simulink model "gm_uz_pmsm_model_6ph_dqxy"  (R2024b)
settings: Solver=FixedStepAuto  StartTime=0.0  StopTime=0.5  RelTol=1e-3
PreLoadFcn:
  | uz_pmsm_model_6ph_dqxy_init_parameter
undefined symbols (not defined in the file or in its folder): friction_coefficient, inertia, k_i_d, k_i_x, k_i_y, k_p_d, k_p_q, k_p_x, k_p_y, L_d, L_q, L_x, L_y, polepair, psi_pm, R_1, setpoint_step, simulate_mechanical, simulate_open_loop, static_friction_torque
libraries: hdlmdlgenlib x5, slpidlib x4
(part 2 of 2)

== system gm_uz_pmsm_model_6ph_dqxy/uz_pmsm_model/Data Type Conversion18 ==
  In1 : Inport
  Data Type Conversion18 : DataTypeConversion  OutDataTypeStr=double  RndMeth=Nearest  SampleTime=1e-08  SaturateOnIntegerOverflow=off
  Data Type Conversion18_pd1 : Delay  DelayLength=3
  Out1 : Outport
  wires:
  In1/1 -> Data Type Conversion18/1
  Data Type Conversion18/1 -> Data Type Conversion18_pd1/1
  Data Type Conversion18_pd1/1 -> Out1/1

== system gm_uz_pmsm_model_6ph_dqxy/uz_pmsm_model/Data Type Conversion19 ==
  In1 : Inport
  Data Type Conversion19 : DataTypeConversion  OutDataTypeStr=double  RndMeth=Nearest  SampleTime=1e-08  SaturateOnIntegerOverflow=off
  Data Type Conversion19_pd1 : Delay  DelayLength=3
  Out1 : Outport
  wires:
  In1/1 -> Data Type Conversion19/1
  Data Type Conversion19/1 -> Data Type Conversion19_pd1/1
  Data Type Conversion19_pd1/1 -> Out1/1

== system gm_uz_pmsm_model_6ph_dqxy/uz_pmsm_model/Data Type Conversion2 ==
  In1 : Inport
  Data Type Conversion2 : DataTypeConversion  OutDataTypeStr=double  RndMeth=Nearest  SampleTime=1e-08  SaturateOnIntegerOverflow=off
  Data Type Conversion2_pd1 : Delay  DelayLength=3
  Out1 : Outport
  wires:
  In1/1 -> Data Type Conversion2/1
  Data Type Conversion2/1 -> Data Type Conversion2_pd1/1
  Data Type Conversion2_pd1/1 -> Out1/1

== system gm_uz_pmsm_model_6ph_dqxy/uz_pmsm_model/Data Type Conversion20 ==
  In1 : Inport
  Data Type Conversion20 : DataTypeConversion  OutDataTypeStr=double  RndMeth=Nearest  SampleTime=1e-08  SaturateOnIntegerOverflow=off
  Data Type Conversion20_pd1 : Delay  DelayLength=3
  Out1 : Outport
  wires:
  In1/1 -> Data Type Conversion20/1
  Data Type Conversion20/1 -> Data Type Conversion20_pd1/1
  Data Type Conversion20_pd1/1 -> Out1/1

== system gm_uz_pmsm_model_6ph_dqxy/uz_pmsm_model/Data Type Conversion21 ==
  In1 : Inport
  Data Type Conversion21 : DataTypeConversion  OutDataTypeStr=single  RndMeth=Nearest  SampleTime=1e-08  SaturateOnIntegerOverflow=off
  Data Type Conversion21_pd1 : Delay  DelayLength=3
  Out1 : Outport
  wires:
  In1/1 -> Data Type Conversion21/1
  Data Type Conversion21/1 -> Data Type Conversion21_pd1/1
  Data Type Conversion21_pd1/1 -> Out1/1

== system gm_uz_pmsm_model_6ph_dqxy/uz_pmsm_model/Data Type Conversion22 ==
  In1 : Inport
  Data Type Conversion22 : DataTypeConversion  OutDataTypeStr=single  RndMeth=Nearest  SampleTime=1e-08  SaturateOnIntegerOverflow=off
  Data Type Conversion22_pd1 : Delay  DelayLength=3
  Out1 : Outport
  wires:
  In1/1 -> Data Type Conversion22/1
  Data Type Conversion22/1 -> Data Type Conversion22_pd1/1
  Data Type Conversion22_pd1/1 -> Out1/1

== system gm_uz_pmsm_model_6ph_dqxy/uz_pmsm_model/Data Type Conversion3 ==
  In1 : Inport
  Data Type Conversion3 : DataTypeConversion  OutDataTypeStr=double  RndMeth=Nearest  SampleTime=1e-08  SaturateOnIntegerOverflow=off
  Data Type Conversion3_pd1 : Delay  DelayLength=3
  Out1 : Outport
  wires:
  In1/1 -> Data Type Conversion3/1
  Data Type Conversion3/1 -> Data Type Conversion3_pd1/1
  Data Type Conversion3_pd1/1 -> Out1/1

== system gm_uz_pmsm_model_6ph_dqxy/uz_pmsm_model/Data Type Conversion4 ==
  In1 : Inport
  Data Type Conversion4 : DataTypeConversion  OutDataTypeStr=double  RndMeth=Nearest  SampleTime=1e-08  SaturateOnIntegerOverflow=off
  Data Type Conversion4_pd1 : Delay  DelayLength=3
  Out1 : Outport
  wires:
  In1/1 -> Data Type Conversion4/1
  Data Type Conversion4/1 -> Data Type Conversion4_pd1/1
  Data Type Conversion4_pd1/1 -> Out1/1

== system gm_uz_pmsm_model_6ph_dqxy/uz_pmsm_model/Data Type Conversion5 ==
  In1 : Inport
  Data Type Conversion5 : DataTypeConversion  OutDataTypeStr=double  RndMeth=Nearest  SampleTime=1e-08  SaturateOnIntegerOverflow=off
  Data Type Conversion5_pd1 : Delay  DelayLength=3
  Out1 : Outport
  wires:
  In1/1 -> Data Type Conversion5/1
  Data Type Conversion5/1 -> Data Type Conversion5_pd1/1
  Data Type Conversion5_pd1/1 -> Out1/1

== system gm_uz_pmsm_model_6ph_dqxy/uz_pmsm_model/Data Type Conversion6 ==
  In1 : Inport
  Data Type Conversion6 : DataTypeConversion  OutDataTypeStr=double  RndMeth=Nearest  SampleTime=1e-08  SaturateOnIntegerOverflow=off
  Data Type Conversion6_pd1 : Delay  DelayLength=3
  Out1 : Outport
  wires:
  In1/1 -> Data Type Conversion6/1
  Data Type Conversion6/1 -> Data Type Conversion6_pd1/1
  Data Type Conversion6_pd1/1 -> Out1/1

== system gm_uz_pmsm_model_6ph_dqxy/uz_pmsm_model/Data Type Conversion7 ==
  In1 : Inport
  Data Type Conversion7 : DataTypeConversion  OutDataTypeStr=double  RndMeth=Nearest  SampleTime=1e-08  SaturateOnIntegerOverflow=off
  Data Type Conversion7_pd1 : Delay  DelayLength=3
  Out1 : Outport
  wires:
  In1/1 -> Data Type Conversion7/1
  Data Type Conversion7/1 -> Data Type Conversion7_pd1/1
  Data Type Conversion7_pd1/1 -> Out1/1

== system gm_uz_pmsm_model_6ph_dqxy/uz_pmsm_model/Data Type Conversion8 ==
  In1 : Inport
  Data Type Conversion8 : DataTypeConversion  OutDataTypeStr=double  RndMeth=Nearest  SampleTime=1e-08  SaturateOnIntegerOverflow=off
  Data Type Conversion8_pd1 : Delay  DelayLength=3
  Out1 : Outport
  wires:
  In1/1 -> Data Type Conversion8/1
  Data Type Conversion8/1 -> Data Type Conversion8_pd1/1
  Data Type Conversion8_pd1/1 -> Out1/1

== system gm_uz_pmsm_model_6ph_dqxy/uz_pmsm_model/Data Type Conversion9 ==
  In1 : Inport
  Data Type Conversion9 : DataTypeConversion  OutDataTypeStr=double  RndMeth=Nearest  SampleTime=1e-08  SaturateOnIntegerOverflow=off
  Data Type Conversion9_pd1 : Delay  DelayLength=3
  Out1 : Outport
  wires:
  In1/1 -> Data Type Conversion9/1
  Data Type Conversion9/1 -> Data Type Conversion9_pd1/1
  Data Type Conversion9_pd1/1 -> Out1/1

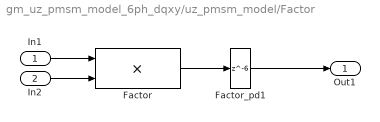
== system gm_uz_pmsm_model_6ph_dqxy/uz_pmsm_model/Factor ==
  In1 : Inport
  In2 : Inport  Port=2
  Factor : Product  Inputs=**  OutDataTypeStr=double  SampleTime=1e-08
  Factor_pd1 : Delay  DelayLength=6
  Out1 : Outport
  wires:
  In1/1 -> Factor/1
  In2/1 -> Factor/2
  Factor/1 -> Factor_pd1/1
  Factor_pd1/1 -> Out1/1

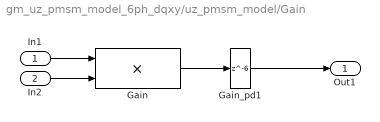
== system gm_uz_pmsm_model_6ph_dqxy/uz_pmsm_model/Gain ==
  In1 : Inport
  In2 : Inport  Port=2
  Gain : Product  Inputs=**  OutDataTypeStr=double  SampleTime=1e-08
  Gain_pd1 : Delay  DelayLength=6
  Out1 : Outport
  wires:
  In1/1 -> Gain/1
  In2/1 -> Gain/2
  Gain/1 -> Gain_pd1/1
  Gain_pd1/1 -> Out1/1

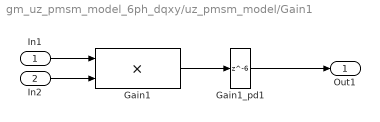
== system gm_uz_pmsm_model_6ph_dqxy/uz_pmsm_model/Gain1 ==
  In1 : Inport
  In2 : Inport  Port=2
  Gain1 : Product  Inputs=**  OutDataTypeStr=double  SampleTime=1e-08
  Gain1_pd1 : Delay  DelayLength=6
  Out1 : Outport
  wires:
  In1/1 -> Gain1/1
  In2/1 -> Gain1/2
  Gain1/1 -> Gain1_pd1/1
  Gain1_pd1/1 -> Out1/1

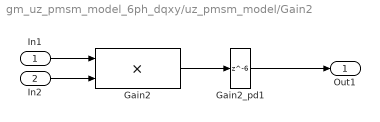
== system gm_uz_pmsm_model_6ph_dqxy/uz_pmsm_model/Gain2 ==
  In1 : Inport
  In2 : Inport  Port=2
  Gain2 : Product  Inputs=**  OutDataTypeStr=double  SampleTime=1e-08
  Gain2_pd1 : Delay  DelayLength=6
  Out1 : Outport
  wires:
  In1/1 -> Gain2/1
  In2/1 -> Gain2/2
  Gain2/1 -> Gain2_pd1/1
  Gain2_pd1/1 -> Out1/1

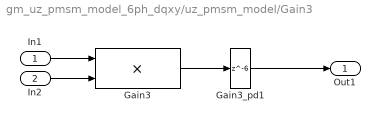
== system gm_uz_pmsm_model_6ph_dqxy/uz_pmsm_model/Gain3 ==
  In1 : Inport
  In2 : Inport  Port=2
  Gain3 : Product  Inputs=**  OutDataTypeStr=double  SampleTime=1e-08
  Gain3_pd1 : Delay  DelayLength=6
  Out1 : Outport
  wires:
  In1/1 -> Gain3/1
  In2/1 -> Gain3/2
  Gain3/1 -> Gain3_pd1/1
  Gain3_pd1/1 -> Out1/1

== system gm_uz_pmsm_model_6ph_dqxy/uz_pmsm_model/Gain4 ==
  In1 : Inport
  In2 : Inport  Port=2
  Gain4 : Product  Inputs=**  OutDataTypeStr=double  SampleTime=1e-08
  Gain4_pd1 : Delay  DelayLength=6
  Out1 : Outport
  wires:
  In1/1 -> Gain4/1
  In2/1 -> Gain4/2
  Gain4/1 -> Gain4_pd1/1
  Gain4_pd1/1 -> Out1/1

== system gm_uz_pmsm_model_6ph_dqxy/uz_pmsm_model/Product ==
  In1 : Inport
  In2 : Inport  Port=2
  Product : Product  Inputs=**  OutDataTypeStr=double  SampleTime=1e-08
  Product_pd1 : Delay  DelayLength=6
  Out1 : Outport
  wires:
  In1/1 -> Product/1
  In2/1 -> Product/2
  Product/1 -> Product_pd1/1
  Product_pd1/1 -> Out1/1

== system gm_uz_pmsm_model_6ph_dqxy/uz_pmsm_model/Product1 ==
  In1 : Inport
  In2 : Inport  Port=2
  Product1 : Product  Inputs=**  OutDataTypeStr=double  SampleTime=1e-08
  Product1_pd1 : Delay  DelayLength=6
  Out1 : Outport
  wires:
  In1/1 -> Product1/1
  In2/1 -> Product1/2
  Product1/1 -> Product1_pd1/1
  Product1_pd1/1 -> Out1/1

== system gm_uz_pmsm_model_6ph_dqxy/uz_pmsm_model/Product10 ==
  In1 : Inport
  In2 : Inport  Port=2
  Product10 : Product  Inputs=**  OutDataTypeStr=double  SampleTime=1e-08
  Product10_pd1 : Delay  DelayLength=6
  Out1 : Outport
  wires:
  In1/1 -> Product10/1
  In2/1 -> Product10/2
  Product10/1 -> Product10_pd1/1
  Product10_pd1/1 -> Out1/1

== system gm_uz_pmsm_model_6ph_dqxy/uz_pmsm_model/Product11 ==
  In1 : Inport
  In2 : Inport  Port=2
  Product11 : Product  Inputs=**  OutDataTypeStr=double  SampleTime=1e-08
  Product11_pd1 : Delay  DelayLength=6
  Out1 : Outport
  wires:
  In1/1 -> Product11/1
  In2/1 -> Product11/2
  Product11/1 -> Product11_pd1/1
  Product11_pd1/1 -> Out1/1

== system gm_uz_pmsm_model_6ph_dqxy/uz_pmsm_model/Product111 ==
  In1 : Inport
  In2 : Inport  Port=2
  Product111 : Product  Inputs=**  OutDataTypeStr=double  SampleTime=1e-08
  Product111_pd1 : Delay  DelayLength=6
  Out1 : Outport
  wires:
  In1/1 -> Product111/1
  In2/1 -> Product111/2
  Product111/1 -> Product111_pd1/1
  Product111_pd1/1 -> Out1/1

== system gm_uz_pmsm_model_6ph_dqxy/uz_pmsm_model/Product12 ==
  In1 : Inport
  In2 : Inport  Port=2
  Product12 : Product  Inputs=**  OutDataTypeStr=double  SampleTime=1e-08
  Product12_pd1 : Delay  DelayLength=6
  Out1 : Outport
  wires:
  In1/1 -> Product12/1
  In2/1 -> Product12/2
  Product12/1 -> Product12_pd1/1
  Product12_pd1/1 -> Out1/1

== system gm_uz_pmsm_model_6ph_dqxy/uz_pmsm_model/Product121 ==
  In1 : Inport
  In2 : Inport  Port=2
  Product121 : Product  Inputs=**  OutDataTypeStr=double  SampleTime=1e-08
  Product121_pd1 : Delay  DelayLength=6
  Out1 : Outport
  wires:
  In1/1 -> Product121/1
  In2/1 -> Product121/2
  Product121/1 -> Product121_pd1/1
  Product121_pd1/1 -> Out1/1

== system gm_uz_pmsm_model_6ph_dqxy/uz_pmsm_model/Product13 ==
  In1 : Inport
  In2 : Inport  Port=2
  Product13 : Product  Inputs=**  OutDataTypeStr=double  SampleTime=1e-08
  Product13_pd1 : Delay  DelayLength=6
  Out1 : Outport
  wires:
  In1/1 -> Product13/1
  In2/1 -> Product13/2
  Product13/1 -> Product13_pd1/1
  Product13_pd1/1 -> Out1/1

== system gm_uz_pmsm_model_6ph_dqxy/uz_pmsm_model/Product2 ==
  In1 : Inport
  In2 : Inport  Port=2
  Product2 : Product  Inputs=**  OutDataTypeStr=double  SampleTime=1e-08
  Product2_pd1 : Delay  DelayLength=6
  Out1 : Outport
  wires:
  In1/1 -> Product2/1
  In2/1 -> Product2/2
  Product2/1 -> Product2_pd1/1
  Product2_pd1/1 -> Out1/1

== system gm_uz_pmsm_model_6ph_dqxy/uz_pmsm_model/Product21 ==
  In1 : Inport
  In2 : Inport  Port=2
  Product21 : Product  Inputs=**  OutDataTypeStr=double  SampleTime=1e-08
  Product21_pd1 : Delay  DelayLength=6
  Out1 : Outport
  wires:
  In1/1 -> Product21/1
  In2/1 -> Product21/2
  Product21/1 -> Product21_pd1/1
  Product21_pd1/1 -> Out1/1

== system gm_uz_pmsm_model_6ph_dqxy/uz_pmsm_model/Product3 ==
  In1 : Inport
  In2 : Inport  Port=2
  Product3 : Product  Inputs=**  OutDataTypeStr=double  SampleTime=1e-08
  Product3_pd1 : Delay  DelayLength=6
  Out1 : Outport
  wires:
  In1/1 -> Product3/1
  In2/1 -> Product3/2
  Product3/1 -> Product3_pd1/1
  Product3_pd1/1 -> Out1/1

== system gm_uz_pmsm_model_6ph_dqxy/uz_pmsm_model/Product31 ==
  In1 : Inport
  In2 : Inport  Port=2
  Product31 : Product  Inputs=**  OutDataTypeStr=double  SampleTime=1e-08
  Product31_pd1 : Delay  DelayLength=6
  Out1 : Outport
  wires:
  In1/1 -> Product31/1
  In2/1 -> Product31/2
  Product31/1 -> Product31_pd1/1
  Product31_pd1/1 -> Out1/1

== system gm_uz_pmsm_model_6ph_dqxy/uz_pmsm_model/Product4 ==
  In1 : Inport
  In2 : Inport  Port=2
  Product4 : Product  Inputs=**  OutDataTypeStr=double  SampleTime=1e-08
  Product4_pd1 : Delay  DelayLength=6
  Out1 : Outport
  wires:
  In1/1 -> Product4/1
  In2/1 -> Product4/2
  Product4/1 -> Product4_pd1/1
  Product4_pd1/1 -> Out1/1

== system gm_uz_pmsm_model_6ph_dqxy/uz_pmsm_model/Product5 ==
  In1 : Inport
  In2 : Inport  Port=2
  Product5 : Product  Inputs=**  OutDataTypeStr=double  SampleTime=1e-08
  Product5_pd1 : Delay  DelayLength=6
  Out1 : Outport
  wires:
  In1/1 -> Product5/1
  In2/1 -> Product5/2
  Product5/1 -> Product5_pd1/1
  Product5_pd1/1 -> Out1/1

== system gm_uz_pmsm_model_6ph_dqxy/uz_pmsm_model/Product6 ==
  In1 : Inport
  In2 : Inport  Port=2
  Product6 : Product  Inputs=**  OutDataTypeStr=double  SampleTime=1e-08
  Product6_pd1 : Delay  DelayLength=6
  Out1 : Outport
  wires:
  In1/1 -> Product6/1
  In2/1 -> Product6/2
  Product6/1 -> Product6_pd1/1
  Product6_pd1/1 -> Out1/1

== system gm_uz_pmsm_model_6ph_dqxy/uz_pmsm_model/Product7 ==
  In1 : Inport
  In2 : Inport  Port=2
  Product7 : Product  Inputs=**  OutDataTypeStr=double  SampleTime=1e-08
  Product7_pd1 : Delay  DelayLength=6
  Out1 : Outport
  wires:
  In1/1 -> Product7/1
  In2/1 -> Product7/2
  Product7/1 -> Product7_pd1/1
  Product7_pd1/1 -> Out1/1

== system gm_uz_pmsm_model_6ph_dqxy/uz_pmsm_model/Product8 ==
  In1 : Inport
  In2 : Inport  Port=2
  Product8 : Product  Inputs=**  OutDataTypeStr=double  SampleTime=1e-08
  Product8_pd1 : Delay  DelayLength=6
  Out1 : Outport
  wires:
  In1/1 -> Product8/1
  In2/1 -> Product8/2
  Product8/1 -> Product8_pd1/1
  Product8_pd1/1 -> Out1/1

== system gm_uz_pmsm_model_6ph_dqxy/uz_pmsm_model/Product9 ==
  In1 : Inport
  In2 : Inport  Port=2
  Product9 : Product  Inputs=**  OutDataTypeStr=double  SampleTime=1e-08
  Product9_pd1 : Delay  DelayLength=6
  Out1 : Outport
  wires:
  In1/1 -> Product9/1
  In2/1 -> Product9/2
  Product9/1 -> Product9_pd1/1
  Product9_pd1/1 -> Out1/1

== system gm_uz_pmsm_model_6ph_dqxy/uz_pmsm_model/Product91 ==
  In1 : Inport
  In2 : Inport  Port=2
  Product91 : Product  Inputs=**  OutDataTypeStr=double  SampleTime=1e-08
  Product91_pd1 : Delay  DelayLength=6
  Out1 : Outport
  wires:
  In1/1 -> Product91/1
  In2/1 -> Product91/2
  Product91/1 -> Product91_pd1/1
  Product91_pd1/1 -> Out1/1

== system gm_uz_pmsm_model_6ph_dqxy/uz_pmsm_model/Sign1 ==
  In1 : Inport
  Sign1 : Signum  SampleTime=1e-08
  Out1 : Outport
  wires:
  In1/1 -> Sign1/1
  Sign1/1 -> Out1/1

== system gm_uz_pmsm_model_6ph_dqxy/uz_pmsm_model/Sum ==
  In1 : Inport
  In2 : Inport  Port=2
  Sum : Sum  Inputs=+-  OutDataTypeStr=double  SampleTime=1e-08
  Sum_pd1 : Delay  DelayLength=6
  Out1 : Outport
  wires:
  In1/1 -> Sum/1
  In2/1 -> Sum/2
  Sum/1 -> Sum_pd1/1
  Sum_pd1/1 -> Out1/1

== system gm_uz_pmsm_model_6ph_dqxy/uz_pmsm_model/Sum1 ==
  In1 : Inport
  In2 : Inport  Port=2
  Sum1 : Sum  Inputs=+-  OutDataTypeStr=double  SampleTime=1e-08
  Sum1_pd1 : Delay  DelayLength=6
  Out1 : Outport
  wires:
  In1/1 -> Sum1/1
  In2/1 -> Sum1/2
  Sum1/1 -> Sum1_pd1/1
  Sum1_pd1/1 -> Out1/1

== system gm_uz_pmsm_model_6ph_dqxy/uz_pmsm_model/Sum1_stage2 ==
  In1 : Inport
  In2 : Inport  Port=2
  Sum1_stage2 : Sum  Inputs=+-  OutDataTypeStr=double  SampleTime=1e-08
  Sum1_stage2_pd1 : Delay  DelayLength=6
  Out1 : Outport
  wires:
  In1/1 -> Sum1_stage2/1
  In2/1 -> Sum1_stage2/2
  Sum1_stage2/1 -> Sum1_stage2_pd1/1
  Sum1_stage2_pd1/1 -> Out1/1

== system gm_uz_pmsm_model_6ph_dqxy/uz_pmsm_model/Sum1_stage3 ==
  In1 : Inport
  In2 : Inport  Port=2
  Sum1_stage3 : Sum  Inputs=+-  OutDataTypeStr=double  SampleTime=1e-08
  Sum1_stage3_pd1 : Delay  DelayLength=6
  Out1 : Outport
  wires:
  In1/1 -> Sum1_stage3/1
  In2/1 -> Sum1_stage3/2
  Sum1_stage3/1 -> Sum1_stage3_pd1/1
  Sum1_stage3_pd1/1 -> Out1/1

== system gm_uz_pmsm_model_6ph_dqxy/uz_pmsm_model/Sum2 ==
  In1 : Inport
  In2 : Inport  Port=2
  Sum2 : Sum  Inputs=+-  OutDataTypeStr=double  SampleTime=1e-08
  Sum2_pd1 : Delay  DelayLength=6
  Out1 : Outport
  wires:
  In1/1 -> Sum2/1
  In2/1 -> Sum2/2
  Sum2/1 -> Sum2_pd1/1
  Sum2_pd1/1 -> Out1/1

== system gm_uz_pmsm_model_6ph_dqxy/uz_pmsm_model/Sum3 ==
  In1 : Inport
  In2 : Inport  Port=2
  Sum3 : Sum  OutDataTypeStr=double  SampleTime=1e-08
  Sum3_pd1 : Delay  DelayLength=6
  Out1 : Outport
  wires:
  In1/1 -> Sum3/1
  In2/1 -> Sum3/2
  Sum3/1 -> Sum3_pd1/1
  Sum3_pd1/1 -> Out1/1

== system gm_uz_pmsm_model_6ph_dqxy/uz_pmsm_model/Sum31 ==
  In1 : Inport
  In2 : Inport  Port=2
  Sum31 : Sum  OutDataTypeStr=double  SampleTime=1e-08
  Sum31_pd1 : Delay  DelayLength=6
  Out1 : Outport
  wires:
  In1/1 -> Sum31/1
  In2/1 -> Sum31/2
  Sum31/1 -> Sum31_pd1/1
  Sum31_pd1/1 -> Out1/1

== system gm_uz_pmsm_model_6ph_dqxy/uz_pmsm_model/Sum32 ==
  In1 : Inport
  In2 : Inport  Port=2
  Sum32 : Sum  OutDataTypeStr=double  SampleTime=1e-08
  Sum32_pd1 : Delay  DelayLength=6
  Out1 : Outport
  wires:
  In1/1 -> Sum32/1
  In2/1 -> Sum32/2
  Sum32/1 -> Sum32_pd1/1
  Sum32_pd1/1 -> Out1/1

== system gm_uz_pmsm_model_6ph_dqxy/uz_pmsm_model/Sum33 ==
  In1 : Inport
  In2 : Inport  Port=2
  Sum33 : Sum  OutDataTypeStr=double  SampleTime=1e-08
  Sum33_pd1 : Delay  DelayLength=6
  Out1 : Outport
  wires:
  In1/1 -> Sum33/1
  In2/1 -> Sum33/2
  Sum33/1 -> Sum33_pd1/1
  Sum33_pd1/1 -> Out1/1

== system gm_uz_pmsm_model_6ph_dqxy/uz_pmsm_model/Sum34 ==
  In1 : Inport
  In2 : Inport  Port=2
  Sum34 : Sum  Inputs=+-  OutDataTypeStr=double  SampleTime=1e-08
  Sum34_pd1 : Delay  DelayLength=6
  Out1 : Outport
  wires:
  In1/1 -> Sum34/1
  In2/1 -> Sum34/2
  Sum34/1 -> Sum34_pd1/1
  Sum34_pd1/1 -> Out1/1

== system gm_uz_pmsm_model_6ph_dqxy/uz_pmsm_model/Sum35 ==
  In1 : Inport
  In2 : Inport  Port=2
  Sum35 : Sum  OutDataTypeStr=double  SampleTime=1e-08
  Sum35_pd1 : Delay  DelayLength=6
  Out1 : Outport
  wires:
  In1/1 -> Sum35/1
  In2/1 -> Sum35/2
  Sum35/1 -> Sum35_pd1/1
  Sum35_pd1/1 -> Out1/1

== system gm_uz_pmsm_model_6ph_dqxy/uz_pmsm_model/Sum3_stage2 ==
  In1 : Inport
  In2 : Inport  Port=2
  Sum3_stage2 : Sum  Inputs=+-  OutDataTypeStr=double  SampleTime=1e-08
  Sum3_stage2_pd1 : Delay  DelayLength=6
  Out1 : Outport
  wires:
  In1/1 -> Sum3_stage2/1
  In2/1 -> Sum3_stage2/2
  Sum3_stage2/1 -> Sum3_stage2_pd1/1
  Sum3_stage2_pd1/1 -> Out1/1

== system gm_uz_pmsm_model_6ph_dqxy/uz_pmsm_model/Sum3_stage3 ==
  In1 : Inport
  In2 : Inport  Port=2
  Sum3_stage3 : Sum  Inputs=+-  OutDataTypeStr=double  SampleTime=1e-08
  Sum3_stage3_pd1 : Delay  DelayLength=6
  Out1 : Outport
  wires:
  In1/1 -> Sum3_stage3/1
  In2/1 -> Sum3_stage3/2
  Sum3_stage3/1 -> Sum3_stage3_pd1/1
  Sum3_stage3_pd1/1 -> Out1/1

== system gm_uz_pmsm_model_6ph_dqxy/uz_pmsm_model/Sum4_stage2 ==
  In1 : Inport
  In2 : Inport  Port=2
  Sum4_stage2 : Sum  OutDataTypeStr=double  SampleTime=1e-08
  Sum4_stage2_pd1 : Delay  DelayLength=6
  Out1 : Outport
  wires:
  In1/1 -> Sum4_stage2/1
  In2/1 -> Sum4_stage2/2
  Sum4_stage2/1 -> Sum4_stage2_pd1/1
  Sum4_stage2_pd1/1 -> Out1/1

== system gm_uz_pmsm_model_6ph_dqxy/uz_pmsm_model/Sum4_stage3 ==
  In1 : Inport
  In2 : Inport  Port=2
  Sum4_stage3 : Sum  Inputs=+-  OutDataTypeStr=double  SampleTime=1e-08
  Sum4_stage3_pd1 : Delay  DelayLength=6
  Out1 : Outport
  wires:
  In1/1 -> Sum4_stage3/1
  In2/1 -> Sum4_stage3/2
  Sum4_stage3/1 -> Sum4_stage3_pd1/1
  Sum4_stage3_pd1/1 -> Out1/1

== system gm_uz_pmsm_model_6ph_dqxy/uz_pmsm_model/Sum5 ==
  In1 : Inport
  In2 : Inport  Port=2
  Sum5 : Sum  OutDataTypeStr=double  SampleTime=1e-08
  Sum5_pd1 : Delay  DelayLength=6
  Out1 : Outport
  wires:
  In1/1 -> Sum5/1
  In2/1 -> Sum5/2
  Sum5/1 -> Sum5_pd1/1
  Sum5_pd1/1 -> Out1/1

== system gm_uz_pmsm_model_6ph_dqxy/uz_pmsm_model/Sum_stage2 ==
  In1 : Inport
  In2 : Inport  Port=2
  Sum_stage2 : Sum  Inputs=+-  OutDataTypeStr=double  SampleTime=1e-08
  Sum_stage2_pd1 : Delay  DelayLength=6
  Out1 : Outport
  wires:
  In1/1 -> Sum_stage2/1
  In2/1 -> Sum_stage2/2
  Sum_stage2/1 -> Sum_stage2_pd1/1
  Sum_stage2_pd1/1 -> Out1/1

== system gm_uz_pmsm_model_6ph_dqxy/uz_pmsm_model/Sum_stage3 ==
  In1 : Inport
  In2 : Inport  Port=2
  Sum_stage3 : Sum  OutDataTypeStr=double  SampleTime=1e-08
  Sum_stage3_pd1 : Delay  DelayLength=6
  Out1 : Outport
  wires:
  In1/1 -> Sum_stage3/1
  In2/1 -> Sum_stage3/2
  Sum_stage3/1 -> Sum_stage3_pd1/1
  Sum_stage3_pd1/1 -> Out1/1
